simulink model "VehCtrlMdel240926_2018b"  (R2019b)
settings: Solver=FixedStepDiscrete  StartTime=0.0  StopTime=10.0  FixedStep=0.0005  RelTol=1e-3  EnableMultiTasking=on
values from neighbouring files (symbols this model uses):
  Ax_OffSet = 0.0    [VehCtrlMdelDictionary.sldd]
  Ay_OffSet = 0.0    [VehCtrlMdelDictionary.sldd]
  Caf = 460.0    [VehCtrlMdelDictionary.sldd]    (also in trqvparameter.m = 460)
  Car = 440.0    [VehCtrlMdelDictionary.sldd]    (also in trqvparameter.m = 440)
  dwf = 1.2    [VehCtrlMdelDictionary.sldd]    (also in trqvparameter.m)
  dwr = 1.2    [VehCtrlMdelDictionary.sldd]    (also in trqvparameter.m)
  h = 0.29    [VehCtrlMdelDictionary.sldd]    (also in trqvparameter.m)
  i1 = 11.4    [VehCtrlMdelDictionary.sldd]    (also in trqvparameter.m)
  i2 = 3.4    [VehCtrlMdelDictionary.sldd]    (also in trqvparameter.m)
  Iz = 105.0    [VehCtrlMdelDictionary.sldd]    (also in trqvparameter.m = 105)
  Kc = 1.0    [VehCtrlMdelDictionary.sldd]    (also in trqvparameter.m = 10)
  Ki = 1.0    [VehCtrlMdelDictionary.sldd]    (also in trqvparameter.m = 20)
  Kp = 2.0    [VehCtrlMdelDictionary.sldd]    (also in trqvparameter.m = 30)
  Ldwf = 1.2    [VehCtrlMdelDictionary.sldd]    (also in trqvparameter.m)
  Ldwr = 1.16    [VehCtrlMdelDictionary.sldd]    (also in trqvparameter.m)
  lf = 0.761    [VehCtrlMdelDictionary.sldd]    (also in trqvparameter.m)
  lr = 0.831    [VehCtrlMdelDictionary.sldd]    (also in trqvparameter.m)
  m = 340.0    [VehCtrlMdelDictionary.sldd]    (also in trqvparameter.m = 340)
  Offset_Angle = 0.0    [VehCtrlMdelDictionary.sldd]
  Qa = 0.1    [VehCtrlMdelDictionary.sldd]    (also in trqvparameter.m)
  Ra = 2.0    [VehCtrlMdelDictionary.sldd]    (also in trqvparameter.m = 2)
  Rt = 0.2    [VehCtrlMdelDictionary.sldd]    (also in trqvparameter.m)
  thr1 = 2.0    [VehCtrlMdelDictionary.sldd]    (also in trqvparameter.m = 2)
  thr2 = 0.5    [VehCtrlMdelDictionary.sldd]    (also in trqvparameter.m)
  thr3 = 0.8    [VehCtrlMdelDictionary.sldd]    (also in trqvparameter.m)
  thr4 = 0.5    [VehCtrlMdelDictionary.sldd]    (also in trqvparameter.m)
  thr5 = -0.5    [VehCtrlMdelDictionary.sldd]    (also in trqvparameter.m)
  TrqRquRate = 0.1    [VehCtrlMdelDictionary.sldd]    (also in trqvparameter.m)
  YawRate_OffSet = 0.0    [VehCtrlMdelDictionary.sldd]
undefined symbols (not defined in the file or in its folder): DiscIntNeverNeededParam, I_AN06_5V, I_AN07_5V, I_AN08_5V, I_AN09_5V, I_SW01_L, I_SW03_L, O_SW12_HS1A, O_SW14_HS1A, PWM3
libraries: simulink x150, ec5744lib x118, canmsglib x18
(part 6 of 6)

== stateflow chart VehCtrlMdel240926_2018b/Input_Processing/Subsystem/WhlSlpageJudgment/Timer3 ==
  state Trigger
    en:
    x = x + 0.01;
    Exit=0;
  state Out
    en:
    Exit=1;
    x=0;
  state InterState
    en:
    x=0;
  Trigger -> Trigger [order 1] : [Trigger&&x<CountTime]
  Trigger -> Out [order 2] : [x>=CountTime]
  (default) -> Trigger
  Out -> Trigger : [~Trigger]
  InterState -> Trigger : [Trigger]
  Trigger -> InterState [order 3] : [x<CountTime&&~Trigger]
  data: Trigger input; CountTime input; Exit output; x local =0

== matlab function VehCtrlMdel240926_2018b/CTRL/MoTrqReq/DYC/载荷转移 ==
  data: ax input; Fz1 output; Fz2 output; Fz3 output; Fz4 output; ay input; h input; lfw input; lrw input; lf input; lr input; m input
function [Fz1,Fz2,Fz3,Fz4] = fcn(ax,ay,h,lfw,lrw,lf,lr,m)
g = 9.8;

Fz1 = (lr/(lf+lr))*(0.5*m*g-m*ay*h/lfw)-0.5*m*ax*h/(lf+lr);
Fz2 = (lr/(lf+lr))*(0.5*m*g+m*ay*h/lfw)-0.5*m*ax*h/(lf+lr);
Fz3 = (lr/(lf+lr))*(0.5*m*g-m*ay*h/lrw)+0.5*m*ax*h/(lf+lr);
Fz4 = (lr/(lf+lr))*(0.5*m*g+m*ay*h/lrw)+0.5*m*ax*h/(lf+lr);

== stateflow chart VehCtrlMdel240926_2018b/Input/key/Timer ==
  state Trigger
    en:
    x = x + 0.01;
    Exit=0;
  state Out
    en:
    Exit=1;
    x=0;
  state InterState
    en:
    x=0;
  Trigger -> Trigger [order 1] : [Trigger&&x<CountTime]
  Trigger -> Out [order 2] : [x>=CountTime]
  (default) -> Trigger
  Out -> Trigger : [~Trigger]
  InterState -> Trigger : [Trigger]
  Trigger -> InterState [order 3] : [x<CountTime&&~Trigger]
  data: Trigger input; CountTime input; Exit output; x local =0

== matlab function VehCtrlMdel240926_2018b/Input_Processing/Function-Call Subsystem/AccBrkPedal/MATLAB Function ==
  data: u input; y output
function y = fcn(u)

y = max(min(-0.4*(u-3060),100),0);
